simulink model "CoffeeReactor_ex3_2"  (R2023b)
settings: Solver=ode4  StartTime=0.0  StopTime=simulationParameters.Tsim  FixedStep=simulationParameters.Tint  RelTol=1e-3
undefined symbols (not defined in the file): ReactorModel_StateUpdate, simulationParameters, u_0
settings Model: Creator=simone  LastModifiedBy=Utente
settings SolverCC: AlgebraicLoopSolver=TrustRegion
settings DataIOCC: SaveOutput=off  SignalLogging=off  DSMLogging=off  SaveTime=off  ReturnWorkspaceOutputs=off
settings DebuggingCC: UnconnectedInputMsg=warning  UnconnectedOutputMsg=warning  UnconnectedLineMsg=warning
settings ModelReferenceCC: EnableRefExpFcnMdlSchedulingChecks=on
settings RTWCC: DLArmComputeVersion=19.05

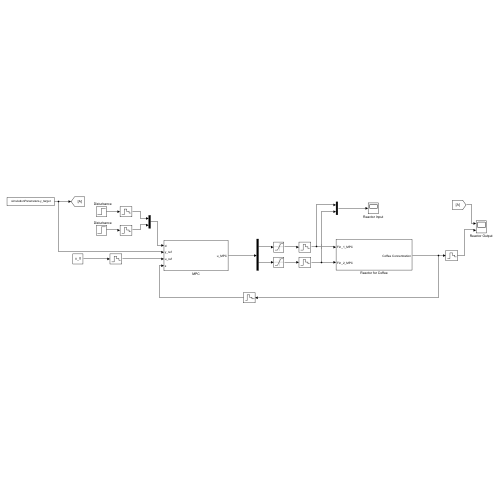
[thumbnail: Simulink's stored preview of the top-level diagram]
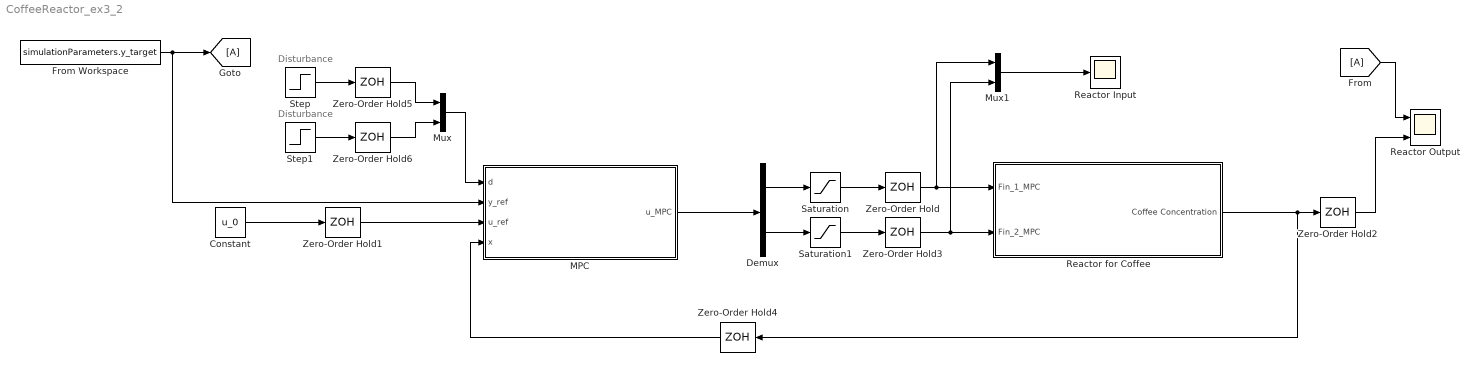
== system CoffeeReactor_ex3_2 ==
  note: Disturbance
  note: Disturbance
  Constant : Constant  Value=u_0
  Demux : Demux  Outputs=2
  From : From
  From Workspace : FromWorkspace  VariableName=simulationParameters.y_target  OutputAfterFinalValue=Holding final value
  Goto : Goto
  MPC : Subsystem
  Mux : Mux  Inputs=2
  Mux1 : Mux  Inputs=2
  Reactor Input : Scope
  Reactor Output : Scope  NumInputPorts=2
  Reactor for Coffee : Subsystem
  Saturation : Saturate  UpperLimit=simulationParameters.Fin1_max  LowerLimit=simulationParameters.Fin1_min
  Saturation1 : Saturate  UpperLimit=simulationParameters.Fin2_max  LowerLimit=simulationParameters.Fin2_min
  Step : Step  Time=simulationParameters.Reactor_parameters.Tdist  After=simulationParameters.Reactor_parameters.Adist  SampleTime=simulationParameters.Ts
  Step1 : Step  Time=simulationParameters.Reactor_parameters.Tdist  After=simulationParameters.Reactor_parameters.Adist  SampleTime=simulationParameters.Ts
  Zero-Order Hold{,1..6} (7 alike) : ZeroOrderHold  SampleTime=simulationParameters.Ts
  wires:
  Reactor for Coffee/1(Coffee Concentration) -> Zero-Order Hold2/1, Zero-Order Hold4/1
  Zero-Order Hold2/1 -> Reactor Output/2
  From/1 -> Reactor Output/1
  From Workspace/1 -> MPC/2(y_ref), Goto/1
  Zero-Order Hold1/1 -> MPC/3(u_ref)
  Step/1 -> Zero-Order Hold5/1
  MPC/1(u_MPC) -> Demux/1
  Demux/1 -> Saturation/1
  Constant/1 -> Zero-Order Hold1/1
  Zero-Order Hold4/1 -> MPC/4(x)
  Saturation/1 -> Zero-Order Hold/1
  Demux/2 -> Saturation1/1
  Zero-Order Hold/1 -> Mux1/1, Reactor for Coffee/1(Fin_1_MPC)
  Saturation1/1 -> Zero-Order Hold3/1
  Zero-Order Hold3/1 -> Mux1/2, Reactor for Coffee/2(Fin_2_MPC)
  Step1/1 -> Zero-Order Hold6/1
  Zero-Order Hold5/1 -> Mux/1
  Zero-Order Hold6/1 -> Mux/2
  Mux/1 -> MPC/1(d)
  Mux1/1 -> Reactor Input/1

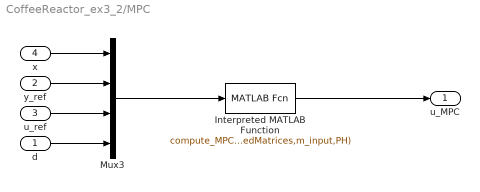
== system CoffeeReactor_ex3_2/MPC ==
  d : Inport
  y_ref : Inport  Port=2
  u_ref : Inport  Port=3
  x : Inport  Port=4
  Interpreted MATLAB Function : MATLABFcn  MATLABFcn=compute_MPC_control(u(1:n),u(n+1:n+p),u(n+p+1:n+p+m_input),u(n+p+m_input+1:end),condensedMatrices,m_input,PH)  OutputDimensions=m_input
  Mux3 : Mux
  u_MPC : Outport
  wires:
  Interpreted MATLAB Function/1 -> u_MPC/1
  Mux3/1 -> Interpreted MATLAB Function/1
  y_ref/1 -> Mux3/2
  u_ref/1 -> Mux3/3
  d/1 -> Mux3/4
  x/1 -> Mux3/1

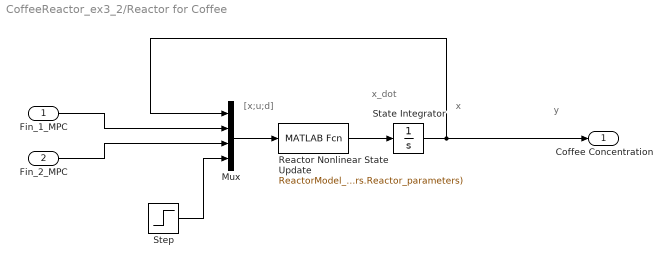
== system CoffeeReactor_ex3_2/Reactor for Coffee ==
  note: y
  note: [x;u;d]
  note: x
  note: x_dot
  Fin_1_MPC : Inport
  Fin_2_MPC : Inport  Port=2
  Mux : Mux
  Reactor Nonlinear State Update : MATLABFcn  MATLABFcn=ReactorModel_StateUpdate(u(1),u(2:3),u(4),simulationParameters.Reactor_parameters)  OutputDimensions=simulationParameters.Reactor_parameters.n
  State Integrator : Integrator  InitialCondition=simulationParameters.Reactor_parameters.x_0
  Step : Step  Time=simulationParameters.Reactor_parameters.Tdist  After=simulationParameters.Reactor_parameters.Adist  SampleTime=0
  Coffee Concentration : Outport
  wires:
  Mux/1 -> Reactor Nonlinear State Update/1
  Fin_2_MPC/1 -> Mux/3
  Reactor Nonlinear State Update/1 -> State Integrator/1
  Fin_1_MPC/1 -> Mux/2
  State Integrator/1 -> Mux/1, Coffee Concentration/1
  Step/1 -> Mux/4
